simulink model "printer"  (R2017b)
settings: Solver=ode45  StartTime=0.0  StopTime=20  RelTol=1e-3  EnableMultiTasking=on
PreLoadFcn:
  | CONSTANTS
  | DEFAULT
  | System
  | Control
InitFcn:
  | CONSTANTS
  | DEFAULT
  | System
  | Control
values from neighbouring files (symbols this model uses):
  Amp0d = [1]    [DEFAULT.m]    (also in System.m = [Amp0d1, Amp0d0]; myattemptOfsystem.m = [Amp0d1 Amp0d0])
  Amp0n = [1]    [DEFAULT.m]    (also in System.m = [Amp0n0]; myattemptOfsystem.m = Amp0n0)
  Amp1d = [Amp1d1, Amp1d0]    [DEFAULT.m]    (also in System.m; SystemHeadless.m = Amp0d; myattemptOfsystem.m = Amp0d)
  Amp1n = [Amp1n0]    [DEFAULT.m]    (also in System.m; SystemHeadless.m = Amp0n; myattemptOfsystem.m = Amp0n)
  AmpSat0 = Big    [DEFAULT.m]    (also in System.m; SystemHeadless.m = q0(NomV); myattemptOfsystem.m)
  AmpSat1 = Big    [DEFAULT.m]    (also in System.m; SystemHeadless.m = AmpSat0; myattemptOfsystem.m)
  BackEMF0 = 0    [DEFAULT.m]    (also in SystemHeadless.m = 1 / q0(SpdK); myattemptOfsystem.m = 1 / BackEMF0_inv)
  BackEMF1 = 0    [DEFAULT.m]    (also in SystemHeadless.m = 1 / q1(SpdK); myattemptOfsystem.m = BackEMF0)
  DegPerRad = 180/pi    (= 57.2957795131)    [CONSTANTS.m]
  Elec0d = [1]    [DEFAULT.m]    (also in SystemHeadless.m = [Elec0d1, Elec0d0]; myattemptOfsystem.m = [Elec0d1 Elec0d0])
  Elec0n = [1]    [DEFAULT.m]    (also in SystemHeadless.m = 1; myattemptOfsystem.m = 1)
  Elec1d = [1]    [DEFAULT.m]    (also in SystemHeadless.m = [Elec1d1, Elec1d0]; myattemptOfsystem.m = Elec0d)
  Elec1n = [1]    [DEFAULT.m]    (also in SystemHeadless.m = 1; myattemptOfsystem.m = 1)
  FB0 = (SensAng * RadPerDeg) / SensV    [Control.m]    (also in DEFAULT.m = 0)
  FB1 = FB0    [Control.m]    (also in DEFAULT.m = 0)
  Height = 200    [CONSTANTS.m]
  JntSat1 = Big    [DEFAULT.m]    (also in SystemHeadless.m = joint_limit; myattemptOfsystem.m)
  Mech0d = [1]    [DEFAULT.m]    (also in SystemHeadless.m = [J_0, B_0, K_0]; myattemptOfsystem.m)
  Mech0n = [1]    [DEFAULT.m]    (also in SystemHeadless.m = [1, 0]; myattemptOfsystem.m)
  Mech1d = [1]    [DEFAULT.m]    (also in SystemHeadless.m = [J_1, B_1, K_1]; myattemptOfsystem.m = [J B K])
  Mech1n = [1]    [DEFAULT.m]    (also in SystemHeadless.m = [1, 0]; myattemptOfsystem.m = [1, 0])
  NomI0 = 1    [DEFAULT.m]
  NomI1 = 1    [DEFAULT.m]
  PID0 = [1 0 0]    [Control.m]    (also in DEFAULT.m)
  PID1 = [1 0 0]    [Control.m]    (also in DEFAULT.m)
  Sens0 = 0    [DEFAULT.m]    (also in SystemHeadless.m = SensV / (SensAng * RadPerDeg); myattemptOfsystem.m)
  Sens1 = 0    [DEFAULT.m]    (also in SystemHeadless.m = SensV / (SensAng * RadPerDeg); myattemptOfsystem.m)
  SensSat0 = Big    [DEFAULT.m]    (also in SystemHeadless.m = SensV; myattemptOfsystem.m)
  SensSat1 = Big    [DEFAULT.m]    (also in SystemHeadless.m = SensV; myattemptOfsystem.m)
  StallI0 = 1    [DEFAULT.m]
  StallI1 = 1    [DEFAULT.m]
  StFric0 = 0    [DEFAULT.m]    (also in SystemHeadless.m = mu_SF * inner_fg; myattemptOfsystem.m)
  TConst0 = 1    [DEFAULT.m]    (also in SystemHeadless.m = q0(TorqueK); myattemptOfsystem.m = MotorParam(TorqueK) * MILLIS_TO)
  TConst1 = 1    [DEFAULT.m]    (also in SystemHeadless.m = q1(TorqueK); myattemptOfsystem.m = TConst0)
undefined symbols (not defined in the file or in its folder): magnitude
libraries: simulink x14, vrlib x1
settings Model: Creator=Leos  LastModifiedBy=Moochster
settings DataIOCC: SaveFormat=Array
settings OptimizationCC: ExpressionDepthLimit=2147483647  LifeSpan=inf
settings DebuggingCC: UnderspecifiedInitializationDetection=Classic  MergeDetectMultiDrivingBlocksExec=none  SolverPrmCheckMsg=warning  FcnCallInpInsideContextMsg=warning  StateNameClashWarn=warning  SFUnexpectedBacktrackingDiag=warning  SFNoUnconditionalDefaultTransitionDiag=warning  SFExecutionAtInitializationDiag=none
settings HardwareCC: ProdBitPerPointer=32  ProdBitPerSizeT=32  ProdBitPerPtrDiffT=32  ProdLargestAtomicFloat=None  ProdIntDivRoundTo=Undefined  ProdEndianess=Unspecified  ProdWordSize=32  ProdHWDeviceType=32-bit Generic
settings ModelReferenceCC: PropagateSignalLabelsOutOfModel=off
settings CodeAppCC: StateflowObjectComments=on
settings GRTTargetCC: TargetLangStandard=C89/C90 (ANSI)  GeneratePreprocessorConditionals=Disable all  CombineOutputUpdateFcns=off  GRTInterface=on
settings ConfigComp: CovMetricSettings=dw  CovHtmlReporting=on  CovSaveCumulativeToWorkspaceVar=on  CovSaveSingleToWorkspaceVar=on  CovExternalEMLEnable=off  CovSFcnEnable=off

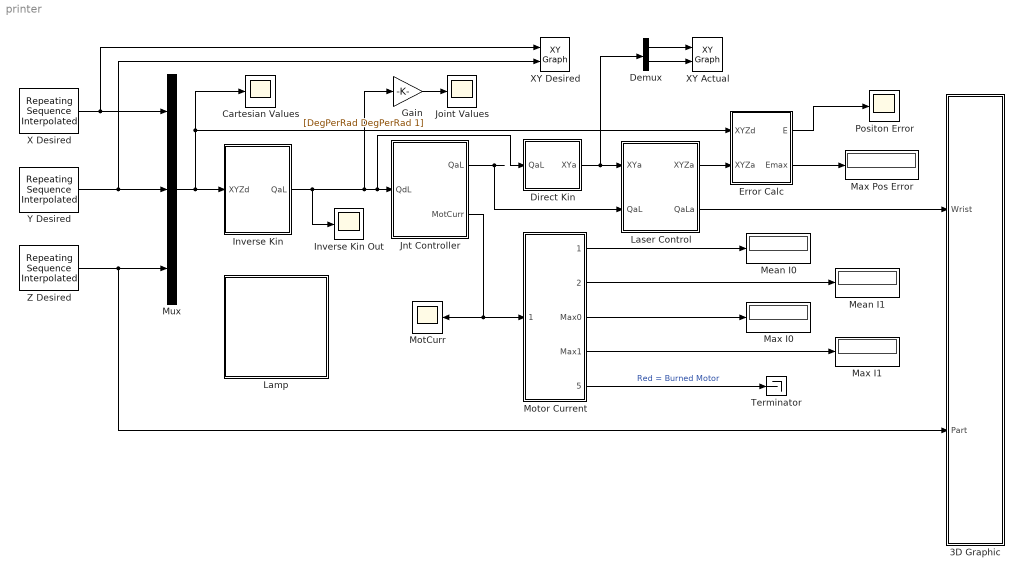
== system printer ==
  3D Graphic : Subsystem
  Cartesian Values : Scope
  Demux : Demux  Outputs=2
  Direct Kin : Subsystem
  Error Calc : Subsystem
  Gain : Gain  Gain=[DegPerRad DegPerRad 1]
  Inverse Kin : Subsystem
  Inverse Kin Out : Scope
  Jnt Controller : Subsystem
  Joint Values : Scope
  Lamp : Subsystem  DialogController=hmiCreateDDGDialog  IsWebBlock=on  mask(MWDashboardBlock){webBlockId=7fcfd6b5-b98b-441a-9880-35fe4990fbef, webBlockType=lamp, ShowInLibBrowser=on, ShowInitialText=on, HMISrcModelName=printer}
      mask prompts: webBlockType "WebBlock Type"; HMISrcModelName "Source Model"
      mask help: SimulinkHMI:dialogs:LampDialogDesc
      mask Help: helpview([docroot '/mapfiles/simulink.map'], 'hmi_lamp')
      mask Display:
      | if strcmp(get_param(bdroot(gcb),'BlockDiagramType'), 'library')
      |     image([(matlabroot) '/toolbox/simulink/hmi/icons/Lamp.png']);
      | end
  Laser Control : Subsystem
  Max I0 : Display
  Max I1 : Display
  Max Pos Error : Display
  Mean I0 : Display
  Mean I1 : Display
  MotCurr : Scope
  Motor Current : Subsystem
  Mux : Mux  Inputs=3
  Positon Error : Scope
  Terminator : Terminator
  X Desired : simulink/Sources/Repeating Sequence Interpolated  OutValues=Xd  TimeValues=Time  LookUpMeth=Interpolation-Use End Values  tsamp=SampleTime  OutMin=[]  OutMax=[]  OutDataTypeStr=double  OutputDataTypeScalingMode=double  OutDataType=fixdt(0,8)  OutScaling=2^-10
  XY Actual : simulink/Sinks/XY Graph  xmin=-125  xmax=125  ymin=-125  ymax=125  st=-1
  XY Desired : simulink/Sinks/XY Graph  xmin=-110  xmax=110  ymin=-110  ymax=110  st=-1
  Y Desired : simulink/Sources/Repeating Sequence Interpolated  OutValues=Yd  TimeValues=Time  LookUpMeth=Interpolation-Use End Values  tsamp=SampleTime  OutMin=[]  OutMax=[]  OutDataTypeStr=double  OutputDataTypeScalingMode=double  OutDataType=fixdt(0,8)  OutScaling=2^-10
  Z Desired : simulink/Sources/Repeating Sequence Interpolated  OutValues=Zd  TimeValues=Time  LookUpMeth=Interpolation-Use End Values  tsamp=SampleTime  OutMin=[]  OutMax=[]  OutDataTypeStr=double  OutputDataTypeScalingMode=double  OutDataType=fixdt(0,8)  OutScaling=2^-10
  wires:
  Inverse Kin/1(QaL) -> Gain/1, Direct Kin/1(QaL), Jnt Controller/1(QdL), Inverse Kin Out/1
  Y Desired/1 -> XY Desired/2, Mux/2
  X Desired/1 -> Mux/1, XY Desired/1
  Demux/2 -> XY Actual/2
  Direct Kin/1(XYa) -> Demux/1, Laser Control/1(XYa)
  Demux/1 -> XY Actual/1
  Z Desired/1 -> 3D Graphic/2(Part), Mux/3
  Jnt Controller/1(QaL) -> Laser Control/2(QaL)
  Laser Control/2(QaLa) -> 3D Graphic/1(Wrist)
  Mux/1 -> Error Calc/1(XYZd), Cartesian Values/1, Inverse Kin/1(XYZd)
  Laser Control/1(XYZa) -> Error Calc/2(XYZa)
  Error Calc/2(Emax) -> Max Pos Error/1
  Error Calc/1(E) -> Positon Error/1
  Jnt Controller/2(MotCurr) -> MotCurr/1, Motor Current/1(MotCurr)
  Motor Current/1(Mean0) -> Mean I0/1
  Motor Current/4(Max1) -> Max I1/1
  Gain/1 -> Joint Values/1
  Motor Current/3(Max0) -> Max I0/1
  Motor Current/2(Mean1) -> Mean I1/1
  Motor Current/5(Burned) -> Terminator/1  "Red = Burned Motor"

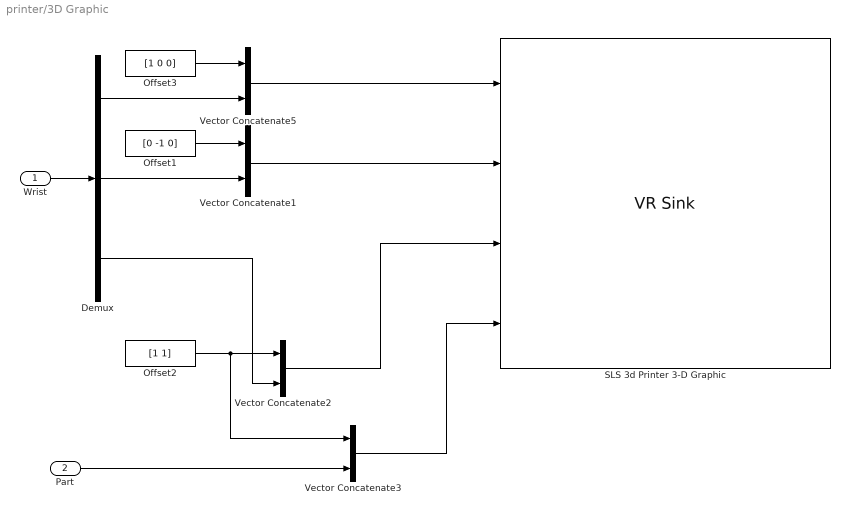
== system printer/3D Graphic ==
  Wrist : Inport
  Part : Inport  Port=2
  Demux : Demux  Outputs=3
  Offset1 : Constant  Value=[0 -1 0]
  Offset2 : Constant  Value=[1 1]
  Offset3 : Constant  Value=[1 0 0]
  SLS 3d Printer 3-D Graphic : vrlib/VR Sink  InstantiateOnLoad=on  SampleTime=.01  ViewEnable=on  RemoteChange=off  RemoteView=off  FieldsWritten=q1.rotation.4.1.1.double#q2.rotation.4.1.1.double#LaserBeam.scale.3.1.1.double#Part.scale.3.1.1.double  WorldFileName=3dPrinter.WRL  AutoView=on  VideoDimensions=[]  AllowVariableSize=off
      settings: SourceProductBaseCode=VR
  Vector Concatenate{1..3,5} (4 alike) : Concatenate
  wires:
  Vector Concatenate1/1 -> SLS 3d Printer 3-D Graphic/2
  Vector Concatenate5/1 -> SLS 3d Printer 3-D Graphic/1
  Demux/1 -> Vector Concatenate5/2
  Demux/2 -> Vector Concatenate1/2
  Offset3/1 -> Vector Concatenate5/1
  Offset1/1 -> Vector Concatenate1/1
  Wrist/1 -> Demux/1
  Offset2/1 -> Vector Concatenate3/1, Vector Concatenate2/1
  Vector Concatenate2/1 -> SLS 3d Printer 3-D Graphic/3
  Part/1 -> Vector Concatenate3/2
  Vector Concatenate3/1 -> SLS 3d Printer 3-D Graphic/4
  Demux/3 -> Vector Concatenate2/2

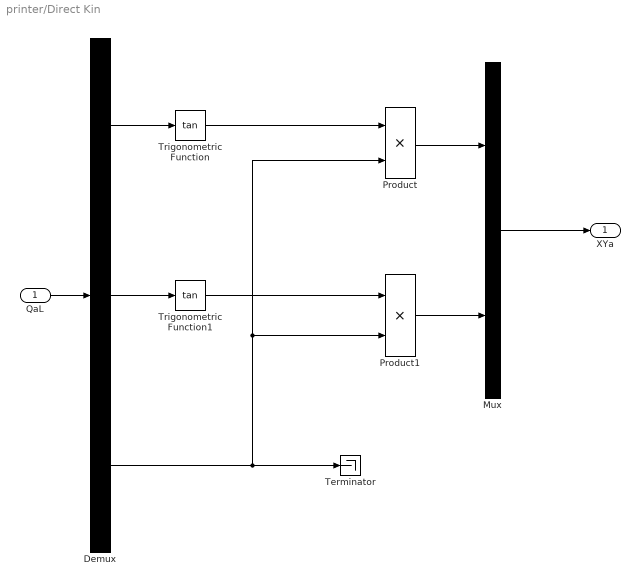
== system printer/Direct Kin ==
  QaL : Inport
  Demux : Demux  Outputs=3
  Mux : Mux  Inputs=2
  Product : Product
  Product1 : Product
  Terminator : Terminator
  Trigonometric Function : Trigonometry  Operator=tan
  Trigonometric Function1 : Trigonometry  Operator=tan
  XYa : Outport
  wires:
  QaL/1 -> Demux/1
  Mux/1 -> XYa/1
  Demux/1 -> Trigonometric Function/1
  Demux/2 -> Trigonometric Function1/1
  Demux/3 -> Product1/2, Product/2, Terminator/1
  Trigonometric Function/1 -> Product/1
  Product/1 -> Mux/1
  Product1/1 -> Mux/2
  Trigonometric Function1/1 -> Product1/1

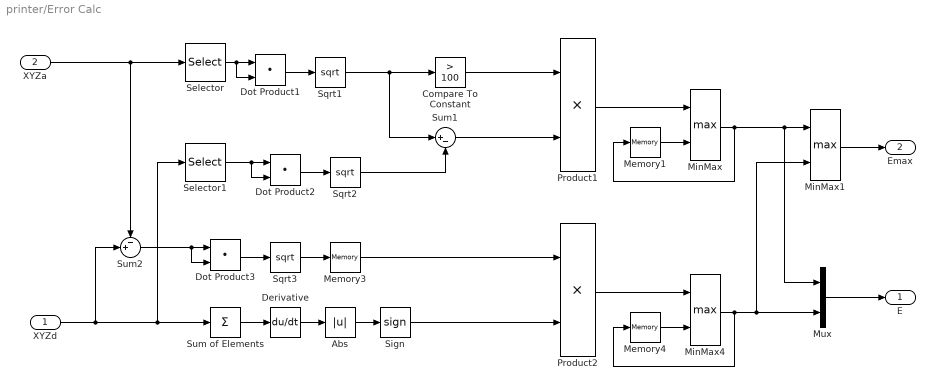
== system printer/Error Calc ==
  XYZd : Inport
  XYZa : Inport  Port=2
  Abs : Abs
  Compare To Constant : simulink/Logic and Bit Operations/Compare To Constant  relop=>  const=100  OutDataTypeStr=boolean
  Derivative : Derivative
  Dot Product1 : DotProduct  InputSameDT=on  OutDataTypeStr=Inherit: Inherit via internal rule
  Dot Product2 : DotProduct  InputSameDT=on  OutDataTypeStr=Inherit: Inherit via internal rule
  Dot Product3 : DotProduct  InputSameDT=on  OutDataTypeStr=Inherit: Inherit via internal rule
  Memory1 : Memory
  Memory3 : Memory
  Memory4 : Memory
  MinMax : MinMax  Function=max  Inputs=2
  MinMax1 : MinMax  Function=max  Inputs=2
  MinMax4 : MinMax  Function=max  Inputs=2
  Mux : Mux  Inputs=2
  Product1 : Product
  Product2 : Product
  Selector : Selector  InputPortWidth=3  IndexOptions=Index vector (dialog)  Indices=[1 2]  OutputSizes=1
  Selector1 : Selector  InputPortWidth=3  IndexOptions=Index vector (dialog)  Indices=[1 2]  OutputSizes=1
  Sign : Signum
  Sqrt1 : Sqrt  SaturateOnIntegerOverflow=on
  Sqrt2 : Sqrt  SaturateOnIntegerOverflow=on
  Sqrt3 : Sqrt  SaturateOnIntegerOverflow=on
  Sum of Elements : Sum  Inputs=+
  Sum1 : Sum  Inputs=|+-
  Sum2 : Sum  Inputs=-+|
  E : Outport
  Emax : Outport  Port=2
  wires:
  XYZd/1 -> Sum2/2, Selector1/1, Sum of Elements/1
  Derivative/1 -> Abs/1
  Abs/1 -> Sign/1
  Sum of Elements/1 -> Derivative/1
  Selector/1 -> Dot Product1/2, Dot Product1/1
  Dot Product1/1 -> Sqrt1/1
  XYZa/1 -> Sum2/1, Selector/1
  Sign/1 -> Product2/2
  Sqrt1/1 -> Sum1/1, Compare To Constant/1
  Product1/1 -> MinMax/1
  Compare To Constant/1 -> Product1/1
  Sum1/1 -> Product1/2
  Memory1/1 -> MinMax/2
  MinMax/1 -> Mux/1, MinMax1/1, Memory1/1
  Memory4/1 -> MinMax4/2
  Product2/1 -> MinMax4/1
  MinMax4/1 -> MinMax1/2, Mux/2, Memory4/1
  MinMax1/1 -> Emax/1
  Mux/1 -> E/1
  Memory3/1 -> Product2/1
  Selector1/1 -> Dot Product2/2, Dot Product2/1
  Dot Product2/1 -> Sqrt2/1
  Sqrt2/1 -> Sum1/2
  Sum2/1 -> Dot Product3/2, Dot Product3/1
  Dot Product3/1 -> Sqrt3/1
  Sqrt3/1 -> Memory3/1

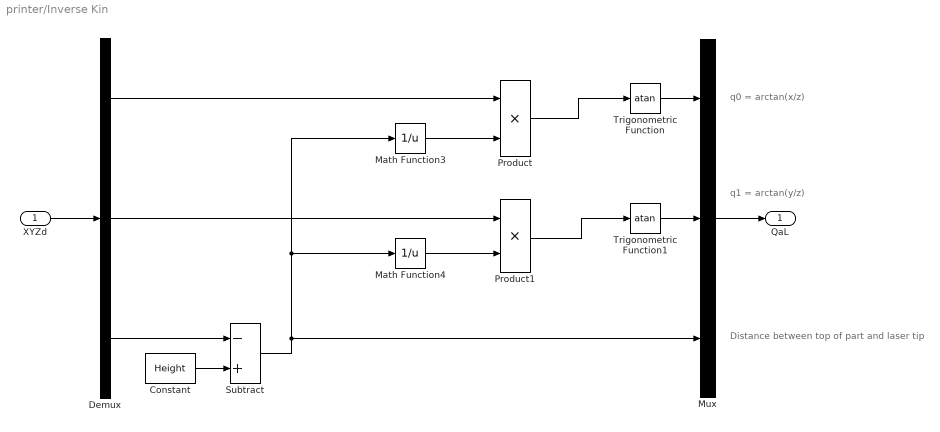
== system printer/Inverse Kin ==
  note: Distance between top of part and laser tip
  note: q0 = arctan(x/z)
  note: q1 = arctan(y/z)
  XYZd : Inport
  Constant : Constant  Value=Height
  Demux : Demux  Outputs=3
  Math Function3 : Math  Operator=reciprocal  SaturateOnIntegerOverflow=on
  Math Function4 : Math  Operator=reciprocal  SaturateOnIntegerOverflow=on
  Mux : Mux  Inputs=3
  Product : Product
  Product1 : Product
  Subtract : Sum  Inputs=-+
  Trigonometric Function : Trigonometry  Operator=atan
  Trigonometric Function1 : Trigonometry  Operator=atan
  QaL : Outport
  wires:
  XYZd/1 -> Demux/1
  Mux/1 -> QaL/1
  Demux/1 -> Product/1
  Demux/2 -> Product1/1
  Demux/3 -> Subtract/1
  Trigonometric Function/1 -> Mux/1
  Trigonometric Function1/1 -> Mux/2
  Constant/1 -> Subtract/2
  Product/1 -> Trigonometric Function/1
  Product1/1 -> Trigonometric Function1/1
  Math Function3/1 -> Product/2
  Math Function4/1 -> Product1/2
  Subtract/1 -> Math Function3/1, Math Function4/1, Mux/3

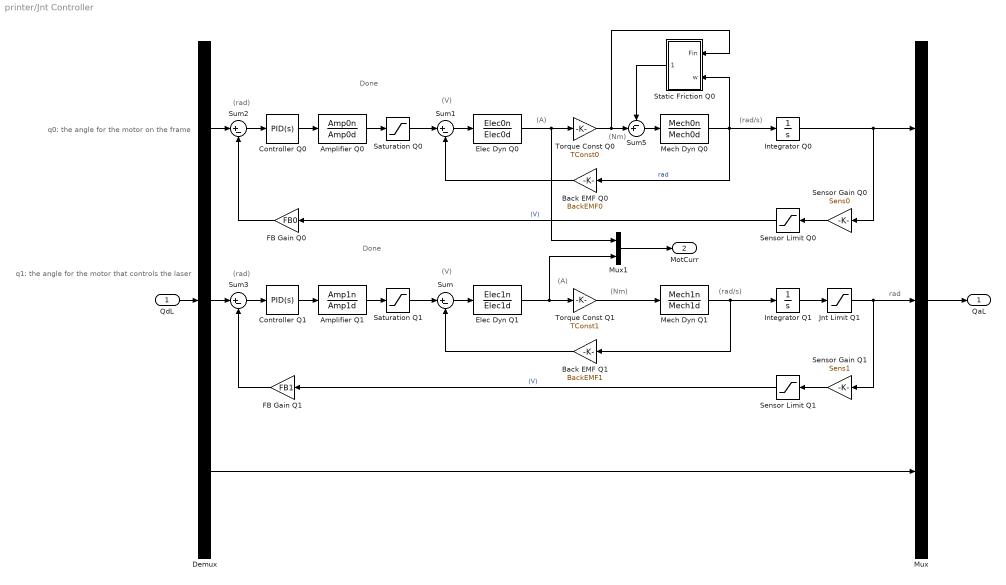
== system printer/Jnt Controller ==
  note: Done
  note: Done
  note: rad
  note: (rad/s)
  note: (V)
  note: (rad)
  note: (A)
  note: (Nm)
  note: (rad/s)
  note: (V)
  note: (rad)
  note: (A)
  note: (Nm)
  note: q0: the angle for the motor on the frame
  note: q1: the angle for the motor that controls the laser
  QdL : Inport
  Amplifier Q0 : TransferFcn  Numerator=Amp0n  Denominator=Amp0d
  Amplifier Q1 : TransferFcn  Numerator=Amp1n  Denominator=Amp1d
  Back EMF Q0 : Gain  Gain=BackEMF0
  Back EMF Q1 : Gain  Gain=BackEMF1
  Controller Q0 : simulink/Continuous/PID Controller  Controller=PID  TimeDomain=Continuous-time  SampleTime=-1  IntegratorMethod=Forward Euler  FilterMethod=Forward Euler  Form=Parallel  UseFilter=on  ControllerParametersSource=internal  P=PID0(1)  I=PID0(2)  D=PID0(3)  N=100  InitialConditionSource=internal  InitialConditionForIntegrator=0  InitialConditionForFilter=0  ExternalReset=none  LimitOutput=off  UpperSaturationLimit=inf  LowerSaturationLimit=-inf  LinearizeAsGain=on  AntiWindupMode=none  Kb=1  TrackingMode=off  Kt=1  PParamMin=[]  PParamMax=[]  IParamMin=[]  IParamMax=[]  DParamMin=[]  DParamMax=[]  NParamMin=[]  NParamMax=[]  KbParamMin=[]  KbParamMax=[]  KtParamMin=[]  KtParamMax=[]  POutMin=[]  POutMax=[]  IOutMin=[]  IOutMax=[]  DOutMin=[]  DOutMax=[]  NOutMin=[]  NOutMax=[]  KbOutMin=[]  KbOutMax=[]  KtOutMin=[]  KtOutMax=[]  IntegratorOutMin=[]  IntegratorOutMax=[]  FilterOutMin=[]  FilterOutMax=[]  SumOutMin=[]  SumOutMax=[]  SumI1OutMin=[]  SumI1OutMax=[]  SumI2OutMin=[]  SumI2OutMax=[]  SumI3OutMin=[]  SumI3OutMax=[]  SumDOutMin=[]  SumDOutMax=[]  SaturationOutMin=[]  SaturationOutMax=[]  IntegratorContinuousStateAttributes=''  IntegratorStateMustResolveToSignalObject=off  IntegratorRTWStateStorageClass=Auto  FilterContinuousStateAttributes=''  FilterStateMustResolveToSignalObject=off  FilterRTWStateStorageClass=Auto  DifferentiatorICPrevScaledInput=0  DifferentiatorOutMin=[]  DifferentiatorOutMax=[]  InitialConditionSetting=State (most efficient)  FilterDiffOutCoefMin=[]  FilterDiffOutCoefMax=[]  SumDenOutMin=[]  SumDenOutMax=[]  SumNumOutMin=[]  SumNumOutMax=[]  ReciprocalOutMin=[]  ReciprocalOutMax=[]  DivideOutMin=[]  DivideOutMax=[]  TunerSelectOption=Transfer Function Based (PID Tuner App)
  Controller Q1 : simulink/Continuous/PID Controller  Controller=PID  TimeDomain=Continuous-time  SampleTime=-1  IntegratorMethod=Forward Euler  FilterMethod=Forward Euler  Form=Parallel  UseFilter=on  ControllerParametersSource=internal  P=PID1(1)  I=PID1(2)  D=PID1(3)  N=100  InitialConditionSource=internal  InitialConditionForIntegrator=0  InitialConditionForFilter=0  ExternalReset=none  LimitOutput=off  UpperSaturationLimit=inf  LowerSaturationLimit=-inf  LinearizeAsGain=on  AntiWindupMode=none  Kb=1  TrackingMode=off  Kt=1  PParamMin=[]  PParamMax=[]  IParamMin=[]  IParamMax=[]  DParamMin=[]  DParamMax=[]  NParamMin=[]  NParamMax=[]  KbParamMin=[]  KbParamMax=[]  KtParamMin=[]  KtParamMax=[]  POutMin=[]  POutMax=[]  IOutMin=[]  IOutMax=[]  DOutMin=[]  DOutMax=[]  NOutMin=[]  NOutMax=[]  KbOutMin=[]  KbOutMax=[]  KtOutMin=[]  KtOutMax=[]  IntegratorOutMin=[]  IntegratorOutMax=[]  FilterOutMin=[]  FilterOutMax=[]  SumOutMin=[]  SumOutMax=[]  SumI1OutMin=[]  SumI1OutMax=[]  SumI2OutMin=[]  SumI2OutMax=[]  SumI3OutMin=[]  SumI3OutMax=[]  SumDOutMin=[]  SumDOutMax=[]  SaturationOutMin=[]  SaturationOutMax=[]  IntegratorContinuousStateAttributes=''  IntegratorStateMustResolveToSignalObject=off  IntegratorRTWStateStorageClass=Auto  FilterContinuousStateAttributes=''  FilterStateMustResolveToSignalObject=off  FilterRTWStateStorageClass=Auto  DifferentiatorICPrevScaledInput=0  DifferentiatorOutMin=[]  DifferentiatorOutMax=[]  InitialConditionSetting=State (most efficient)  FilterDiffOutCoefMin=[]  FilterDiffOutCoefMax=[]  SumDenOutMin=[]  SumDenOutMax=[]  SumNumOutMin=[]  SumNumOutMax=[]  ReciprocalOutMin=[]  ReciprocalOutMax=[]  DivideOutMin=[]  DivideOutMax=[]  TunerSelectOption=Transfer Function Based (PID Tuner App)
  Demux : Demux  Outputs=3
  Elec Dyn Q0 : TransferFcn  Numerator=Elec0n  Denominator=Elec0d
  Elec Dyn Q1 : TransferFcn  Numerator=Elec1n  Denominator=Elec1d
  FB Gain Q0 : Gain  Gain=FB0
  FB Gain Q1 : Gain  Gain=FB1
  Integrator Q0 : Integrator
  Integrator Q1 : Integrator
  Jnt Limit Q1 : Saturate  UpperLimit=JntSat1  LowerLimit=-JntSat1
  Mech Dyn Q0 : TransferFcn  Numerator=Mech0n  Denominator=Mech0d
  Mech Dyn Q1 : TransferFcn  Numerator=Mech1n  Denominator=Mech1d
  Mux : Mux  Inputs=3
  Mux1 : Mux  Inputs=2
  Saturation Q0 : Saturate  UpperLimit=AmpSat0  LowerLimit=-AmpSat0
  Saturation Q1 : Saturate  UpperLimit=AmpSat1  LowerLimit=-AmpSat1
  Sensor Gain Q0 : Gain  Gain=Sens0
  Sensor Gain Q1 : Gain  Gain=Sens1
  Sensor Limit Q0 : Saturate  UpperLimit=SensSat0  LowerLimit=-SensSat0
  Sensor Limit Q1 : Saturate  UpperLimit=SensSat1  LowerLimit=-SensSat1
  Static Friction Q0 : Subsystem
  Sum{,1..3} (4 alike) : Sum  Inputs=|+-
  Sum5 : Sum  Inputs=-+|
  Torque Const Q0 : Gain  Gain=TConst0
  Torque Const Q1 : Gain  Gain=TConst1
  QaL : Outport
  MotCurr : Outport  Port=2
  wires:
  QdL/1 -> Demux/1
  Mux/1 -> QaL/1
  Controller Q1/1 -> Amplifier Q1/1
  Sum/1 -> Elec Dyn Q1/1
  Sum3/1 -> Controller Q1/1
  Elec Dyn Q1/1 -> Mux1/2, Torque Const Q1/1
  Amplifier Q1/1 -> Saturation Q1/1
  Saturation Q1/1 -> Sum/1
  Back EMF Q1/1 -> Sum/2
  Sensor Gain Q1/1 -> Sensor Limit Q1/1
  Controller Q0/1 -> Amplifier Q0/1
  Sum1/1 -> Elec Dyn Q0/1
  Sum2/1 -> Controller Q0/1
  Elec Dyn Q0/1 -> Torque Const Q0/1, Mux1/1
  Amplifier Q0/1 -> Saturation Q0/1
  Saturation Q0/1 -> Sum1/1
  Back EMF Q0/1 -> Sum1/2
  Sensor Gain Q0/1 -> Sensor Limit Q0/1
  Sum5/1 -> Mech Dyn Q0/1
  Jnt Limit Q1/1 -> Mux/2, Sensor Gain Q1/1
  Demux/1 -> Sum2/1
  Demux/3 -> Mux/3
  Demux/2 -> Sum3/1
  FB Gain Q0/1 -> Sum2/2
  FB Gain Q1/1 -> Sum3/2
  Static Friction Q0/1(Fout) -> Sum5/1
  Torque Const Q1/1 -> Mech Dyn Q1/1
  Mux1/1 -> MotCurr/1
  Sensor Limit Q1/1 -> FB Gain Q1/1  "(V)"
  Sensor Limit Q0/1 -> FB Gain Q0/1  "(V)"
  Mech Dyn Q0/1 -> Static Friction Q0/2(w), Integrator Q0/1, Back EMF Q0/1  "rad"
  Integrator Q0/1 -> Sensor Gain Q0/1, Mux/1
  Integrator Q1/1 -> Jnt Limit Q1/1
  Torque Const Q0/1 -> Static Friction Q0/1(Fin), Sum5/2
  Mech Dyn Q1/1 -> Integrator Q1/1, Back EMF Q1/1

== system printer/Lamp ==

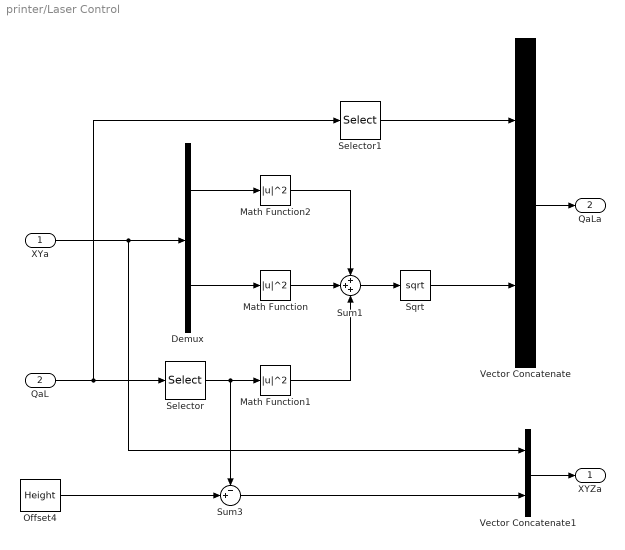
== system printer/Laser Control ==
  XYa : Inport
  QaL : Inport  Port=2
  Demux : Demux  Outputs=2
  Math Function : Math  Operator=magnitude^2  SaturateOnIntegerOverflow=on
  Math Function1 : Math  Operator=magnitude^2  SaturateOnIntegerOverflow=on
  Math Function2 : Math  Operator=magnitude^2  SaturateOnIntegerOverflow=on
  Offset4 : Constant  Value=Height
  Selector : Selector  InputPortWidth=3  IndexOptions=Index vector (dialog)  Indices=3  OutputSizes=1
  Selector1 : Selector  InputPortWidth=3  IndexOptions=Index vector (dialog)  Indices=[1 2]  OutputSizes=1
  Sqrt : Sqrt  SaturateOnIntegerOverflow=on
  Sum1 : Sum  Inputs=+++
  Sum3 : Sum  Inputs=-+|
  Vector Concatenate : Concatenate
  Vector Concatenate1 : Concatenate
  XYZa : Outport
  QaLa : Outport  Port=2
  wires:
  Demux/2 -> Math Function/1
  Demux/1 -> Math Function2/1
  Sqrt/1 -> Vector Concatenate/2
  Math Function2/1 -> Sum1/1
  Math Function/1 -> Sum1/2
  Math Function1/1 -> Sum1/3
  Sum1/1 -> Sqrt/1
  QaL/1 -> Selector1/1, Selector/1
  XYa/1 -> Vector Concatenate1/1, Demux/1
  Selector/1 -> Math Function1/1, Sum3/1
  Selector1/1 -> Vector Concatenate/1
  Vector Concatenate/1 -> QaLa/1
  Vector Concatenate1/1 -> XYZa/1
  Sum3/1 -> Vector Concatenate1/2
  Offset4/1 -> Sum3/2

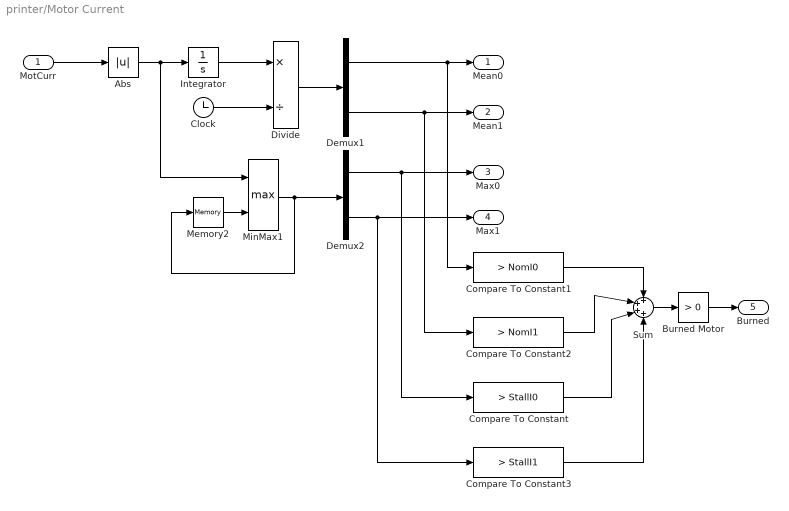
== system printer/Motor Current ==
  MotCurr : Inport
  Abs : Abs
  Burned Motor : simulink/Logic and Bit Operations/Compare To Zero  relop=>  OutDataTypeStr=boolean
  Clock : Clock
  Compare To Constant : simulink/Logic and Bit Operations/Compare To Constant  relop=>  const=StallI0  OutDataTypeStr=boolean
  Compare To Constant1 : simulink/Logic and Bit Operations/Compare To Constant  relop=>  const=NomI0  OutDataTypeStr=boolean
  Compare To Constant2 : simulink/Logic and Bit Operations/Compare To Constant  relop=>  const=NomI1  OutDataTypeStr=boolean
  Compare To Constant3 : simulink/Logic and Bit Operations/Compare To Constant  relop=>  const=StallI1  OutDataTypeStr=boolean
  Demux1 : Demux  Outputs=2
  Demux2 : Demux  Outputs=2
  Divide : Product  Inputs=*/
  Integrator : Integrator
  Memory2 : Memory
  MinMax1 : MinMax  Function=max  Inputs=2
  Sum : Sum  Inputs=++++
  Mean0 : Outport
  Mean1 : Outport  Port=2
  Max0 : Outport  Port=3
  Max1 : Outport  Port=4
  Burned : Outport  Port=5
  wires:
  Demux1/1 -> Compare To Constant1/1, Mean0/1
  MotCurr/1 -> Abs/1
  Integrator/1 -> Divide/1
  Clock/1 -> Divide/2
  Divide/1 -> Demux1/1
  Abs/1 -> MinMax1/1, Integrator/1
  Demux2/1 -> Compare To Constant/1, Max0/1
  Demux1/2 -> Compare To Constant2/1, Mean1/1
  Demux2/2 -> Compare To Constant3/1, Max1/1
  Compare To Constant1/1 -> Sum/1
  Compare To Constant3/1 -> Sum/4
  Compare To Constant/1 -> Sum/3
  Compare To Constant2/1 -> Sum/2
  Memory2/1 -> MinMax1/2
  MinMax1/1 -> Demux2/1, Memory2/1
  Burned Motor/1 -> Burned/1
  Sum/1 -> Burned Motor/1

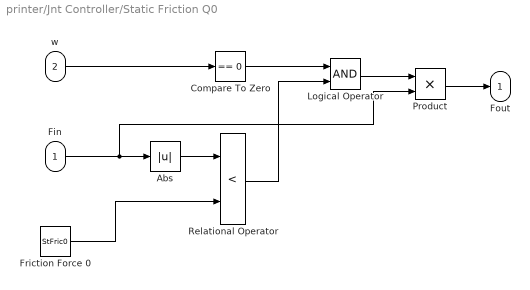
== system printer/Jnt Controller/Static Friction Q0 ==
  Fin : Inport
  w : Inport  Port=2
  Abs : Abs
  Compare To Zero : simulink/Logic and Bit Operations/Compare To Zero  relop===  OutDataTypeStr=boolean
  Friction Force 0 : Constant  Value=StFric0
  Logical Operator : Logic  AllPortsSameDT=off  OutDataTypeStr=boolean
  Product : Product
  Relational Operator : RelationalOperator  Operator=<  OutDataTypeStr=boolean  RndMeth=Simplest
  Fout : Outport
  wires:
  Friction Force 0/1 -> Relational Operator/2
  Product/1 -> Fout/1
  Compare To Zero/1 -> Logical Operator/1
  Relational Operator/1 -> Logical Operator/2
  Logical Operator/1 -> Product/1
  Fin/1 -> Product/2, Abs/1
  w/1 -> Compare To Zero/1
  Abs/1 -> Relational Operator/1
